simulink library "VehicleBody"  (R2021b)
settings: Solver=VariableStepAuto  StartTime=0.0  StopTime=10.0  RelTol=1e-3
undefined symbols (not defined in the file or in its folder): g, h, r_wheel, rho
settings Model: Creator=dadikozyanaa  LastModifiedBy=dadikozyanaa

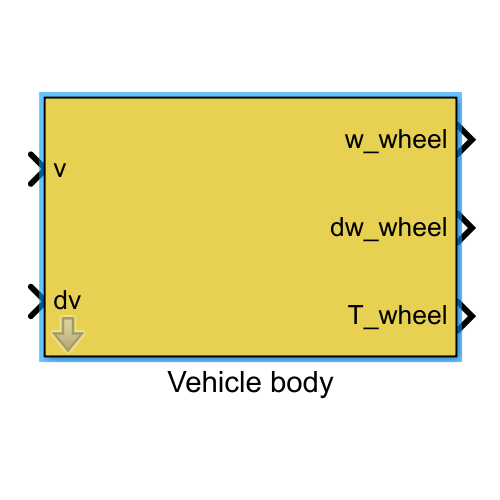
[thumbnail: Simulink's stored preview of the top-level diagram]
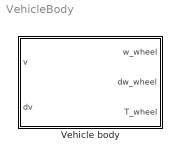
== system VehicleBody ==
  Vehicle body : Subsystem  mask(Vehicle body){m_f=750, mt2m_f=5, A_f=1.8, d_wheel=0.5, cw=0.22, mu=0.008, f_r=0.6, slope_bool=off}
      mask prompts: m_f "Total vehicle mass [kg]:"; mt2m_f "Rotating mass [%]:"; A_f "Vehicle cross section [m2]:"; d_wheel "Wheel diameter [m]:"; cw "Air drag coefficient [-]:"; mu "Rolling resistance coefficient [-]:"; f_r "Regenerative brake fraction [-]:"; slope_bool "Include road slope"
      mask help:
      | This block computes the power required from the vehicle.
      |
      | Input:
      | =====
      | 	v	Speed [m/s]
      | 	dv	Acceleration [m/s^2]
      | 	slope	Road slope [rad] (optional)
      |
      | Output:
      | ======
      | 	w_wheel	Speed of the wheel [rad/s]
      | 	dw_wheel	Acceleration of the wheel [rad/s^2]
      | 	T_wheel	Torque on the wheel [Nm]
      mask init:
      | init_vehicle;
      | %%
      | slope = find_system(gcb, 'LookUnderMasks','on', 'FollowLinks','on', 'Name','slope');
      | %%
      | if(slope_bool)
      |     if isempty(slope)
      |         delete_line(gcb,'Constant_slope/1','goto_slope/1');
      |         delete_block([gcb,'/Constant_slope']);
      |         add_block('built-in/Inport',[gcb,'/slope']);
      |         set_param([gcb,'/slope'],'Position',[830 325 860 355])
      |         add_line(gcb,['slope/1'],['goto_slope/1']);
      |     end
      | else
      |     if ~isempty(slope)
      |         delete_line(gcb,['slope/1'],['goto_slope/1']);
      |         delete_block(slope);
      |         add_block('simulink/Commonly Used Blocks/Constant',[gcb,'/Constant_slope']);
      |         set_param([gcb,'/Constant_slope'],'value','0');
      |         set_param([gcb,'/Constant_slope'],'Position',[830 325 860 355])
      |         add_line(gcb,'Constant_slope/1','goto_slope/1');
      |     end
      | end
      mask DialogControl Container3 Prompt: Optional settings

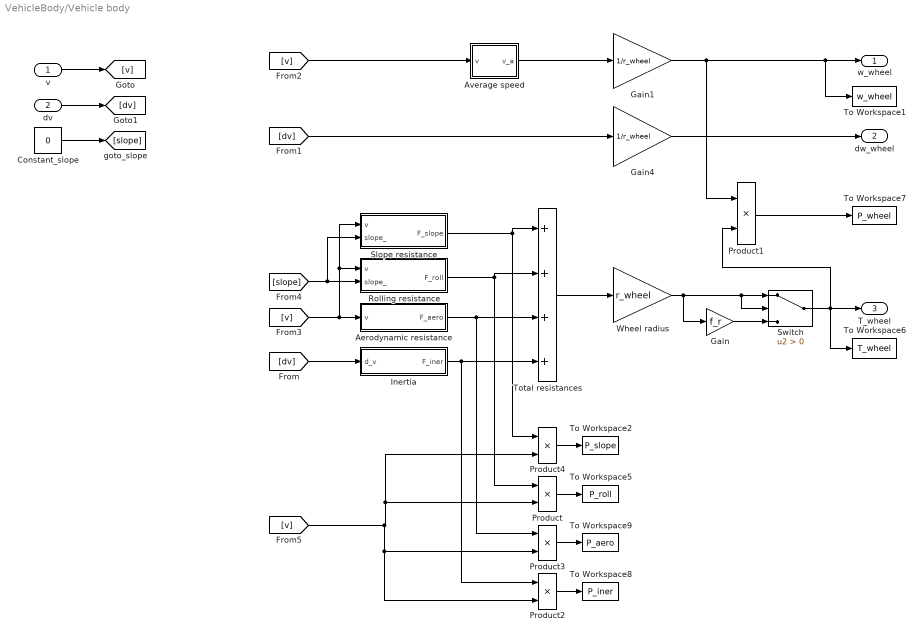
== system VehicleBody/Vehicle body ==
  v : Inport
  dv : Inport  Port=2
  Aerodynamic resistance : Subsystem
  Average speed : Subsystem
  Constant_slope : Constant  Value=0
  Gain : Gain  Gain=f_r
  Gain1 : Gain  Gain=1/r_wheel  SaturateOnIntegerOverflow=on  OutDataTypeStr=Inherit: Same as input  ParamDataTypeStr=Inherit: Same as input
  Gain4 : Gain  Gain=1/r_wheel  SaturateOnIntegerOverflow=on  OutDataTypeStr=Inherit: Same as input  ParamDataTypeStr=Inherit: Same as input
  Inertia : Subsystem
  Product{,1..4} (5 alike) : Product  InputSameDT=on  RndMeth=Zero  SaturateOnIntegerOverflow=on  OutDataTypeStr=Inherit: Same as first input
  Rolling resistance : Subsystem
  Slope resistance : Subsystem
  Switch : Switch  Criteria=u2 > Threshold
  To Workspace1 : ToWorkspace  VariableName=w_wheel  SampleTime=-1
  To Workspace2 : ToWorkspace  VariableName=P_slope  SampleTime=-1
  To Workspace5 : ToWorkspace  VariableName=P_roll  SampleTime=-1
  To Workspace6 : ToWorkspace  VariableName=T_wheel  SampleTime=-1
  To Workspace7 : ToWorkspace  VariableName=P_wheel  SampleTime=-1
  To Workspace8 : ToWorkspace  VariableName=P_iner  SampleTime=-1
  To Workspace9 : ToWorkspace  VariableName=P_aero  SampleTime=-1
  Total resistances : Sum  Inputs=++++  InputSameDT=on  SaturateOnIntegerOverflow=on  OutDataTypeStr=Inherit: Same as first input
  Wheel radius : Gain  Gain=r_wheel  SaturateOnIntegerOverflow=on  OutDataTypeStr=Inherit: Same as input  ParamDataTypeStr=Inherit: Same as input
  w_wheel : Outport  InitialOutput=0
  dw_wheel : Outport  Port=2  InitialOutput=0
  T_wheel : Outport  Port=3  InitialOutput=0
  wires:
  dv/1 -> [dv]
  Inertia/1(F_iner) -> Product2/1, Total resistances/4
  Product1/1 -> To Workspace7/1
  Product4/1 -> To Workspace2/1
  Rolling resistance/1(F_roll) -> Total resistances/2, Product/1
  [v] -> Slope resistance/1(v), Rolling resistance/1(v), Aerodynamic resistance/1(v)
  [v] -> Product3/2, Product2/2, Product/2, Product4/2
  [v] -> Average speed/1(v)
  Aerodynamic resistance/1(F_aero) -> Product3/1, Total resistances/3
  Wheel radius/1 -> Gain/1, Switch/2, Switch/1
  Slope resistance/1(F_slope) -> Total resistances/1, Product4/1
  Product/1 -> To Workspace5/1
  Total resistances/1 -> Wheel radius/1
  [dv] -> Gain4/1
  Gain4/1 -> dw_wheel/1
  Average speed/1(v_a) -> Gain1/1
  Product2/1 -> To Workspace8/1
  v/1 -> [v]
  Product3/1 -> To Workspace9/1
  Gain1/1 -> Product1/1, w_wheel/1, To Workspace1/1
  [dv] -> Inertia/1(d_v)
  [slope] -> Slope resistance/2(slope_), Rolling resistance/2(slope_)
  Constant_slope/1 -> [slope]
  Gain/1 -> Switch/3
  Switch/1 -> Product1/2, To Workspace6/1, T_wheel/1

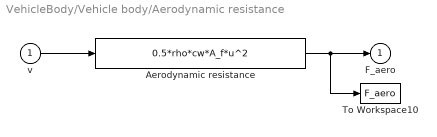
== system VehicleBody/Vehicle body/Aerodynamic resistance ==
  v : Inport
  Aerodynamic resistance : Fcn  Expr=0.5*rho*cw*A_f*u^2
  To Workspace10 : ToWorkspace  VariableName=F_aero  SampleTime=-1
  F_aero : Outport  InitialOutput=0
  wires:
  v/1 -> Aerodynamic resistance/1
  Aerodynamic resistance/1 -> F_aero/1, To Workspace10/1

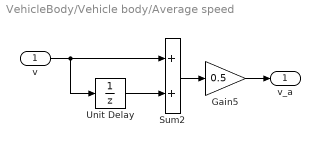
== system VehicleBody/Vehicle body/Average speed ==
  v : Inport
  Gain5 : Gain  Gain=0.5  SaturateOnIntegerOverflow=on  OutDataTypeStr=Inherit: Same as input  ParamDataTypeStr=Inherit: Same as input
  Sum2 : Sum  InputSameDT=on  SaturateOnIntegerOverflow=on  OutDataTypeStr=Inherit: Same as first input
  Unit Delay : UnitDelay  SampleTime=h
  v_a : Outport  InitialOutput=0
  wires:
  Unit Delay/1 -> Sum2/2
  Sum2/1 -> Gain5/1
  Gain5/1 -> v_a/1
  v/1 -> Sum2/1, Unit Delay/1

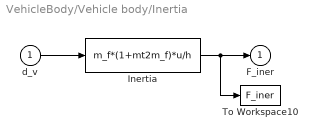
== system VehicleBody/Vehicle body/Inertia ==
  d_v : Inport
  Inertia : Fcn  Expr=m_f*(1+mt2m_f)*u/h
  To Workspace10 : ToWorkspace  VariableName=F_iner  SampleTime=-1
  F_iner : Outport  InitialOutput=0
  wires:
  Inertia/1 -> F_iner/1, To Workspace10/1
  d_v/1 -> Inertia/1

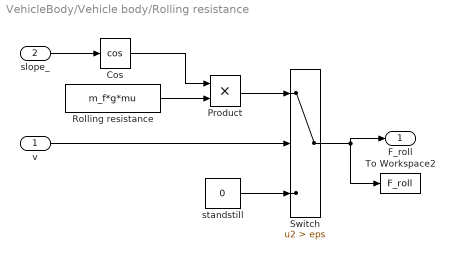
== system VehicleBody/Vehicle body/Rolling resistance ==
  v : Inport
  slope_ : Inport  Port=2
  Cos : Trigonometry  Operator=cos  OutputSignalType=real
  Product : Product
  Rolling resistance : Constant  Value=m_f*g*mu
  Switch : Switch  Criteria=u2 > Threshold  Threshold=eps
  To Workspace2 : ToWorkspace  VariableName=F_roll  SampleTime=-1
  standstill : Constant  Value=0
  F_roll : Outport
  wires:
  Switch/1 -> To Workspace2/1, F_roll/1
  v/1 -> Switch/2
  standstill/1 -> Switch/3
  slope_/1 -> Cos/1
  Cos/1 -> Product/1
  Rolling resistance/1 -> Product/2
  Product/1 -> Switch/1

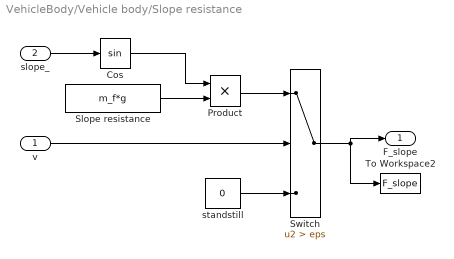
== system VehicleBody/Vehicle body/Slope resistance ==
  v : Inport
  slope_ : Inport  Port=2
  Cos : Trigonometry  OutputSignalType=real
  Product : Product
  Slope resistance : Constant  Value=m_f*g
  Switch : Switch  Criteria=u2 > Threshold  Threshold=eps
  To Workspace2 : ToWorkspace  VariableName=F_slope  SampleTime=-1
  standstill : Constant  Value=0
  F_slope : Outport
  wires:
  Switch/1 -> To Workspace2/1, F_slope/1
  v/1 -> Switch/2
  standstill/1 -> Switch/3
  slope_/1 -> Cos/1
  Cos/1 -> Product/1
  Slope resistance/1 -> Product/2
  Product/1 -> Switch/1
